simulink model "SPWM_Three_Phase_Three_Level_Inverter"  (R2022a)
settings: Solver=ode4  StartTime=0.0  StopTime=1  FixedStep=1e-5  RelTol=1e-3
libraries: spsIGBTDiodeLib x12, simulink x6, spsSeriesRLCBranchLib x3, spsDCVoltageSourceLib x1, spsGroundLib x1, spsThreePhaseVIMeasurementLib x1, spspowerguiLib x1
settings Model: Creator=nikos  LastModifiedBy=nikos

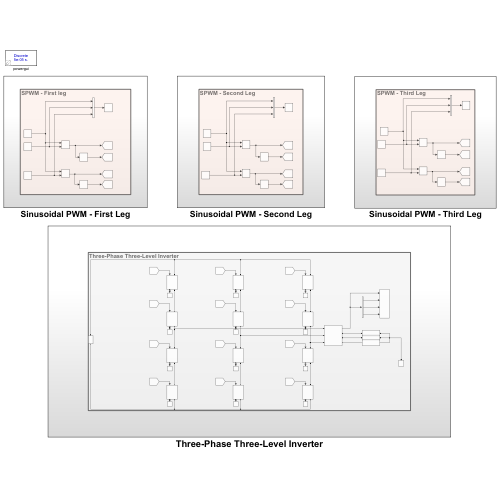
[thumbnail: Simulink's stored preview of the top-level diagram]
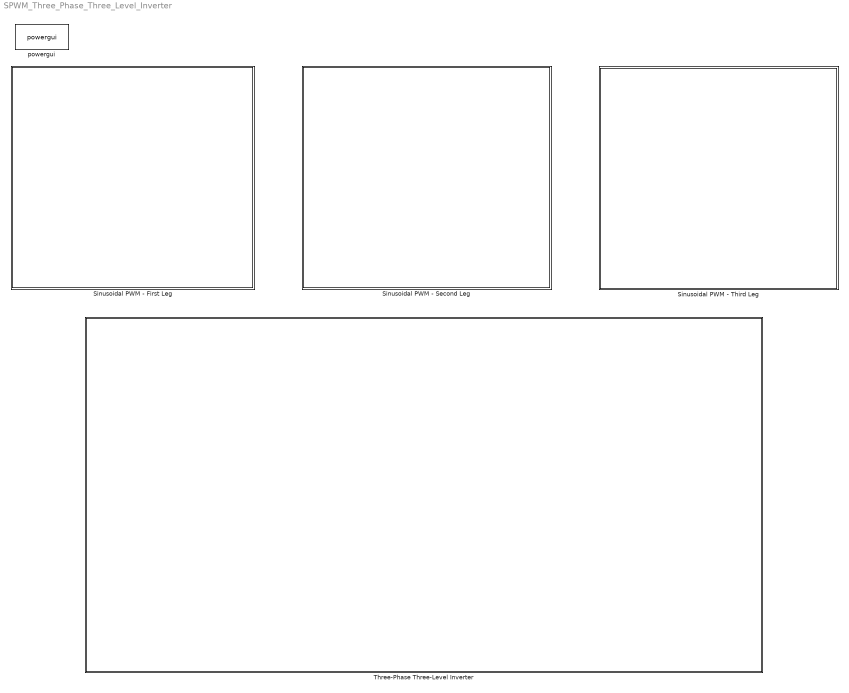
== system SPWM_Three_Phase_Three_Level_Inverter ==
  Sinusoidal PWM - First Leg : Subsystem
  Sinusoidal PWM - Second Leg : Subsystem
  Sinusoidal PWM - Third Leg : Subsystem
  Three-Phase Three-Level Inverter : Subsystem
  powergui : spspowerguiLib/powergui  Priority=1  SimulationMode=Discrete  SampleTime=50e-6  frequency=60  Iterations=50  frequencyindice=0  Pbase=100e6  ErrMax=1e-4  UnitsV=kV  UnitsW=MW  buscounter=0  FunctionMessages=off  echomessages=off  EnableUseOfTLC=off  CurrentSourceSwitches=off  DisableSnubberDevices=off  DisableRonSwitches=off  DisableVfSwitches=off  DisplayEquations=off  AutomaticDiscreteSolvers=off  SolverType=Tustin/Backward Euler (TBE)  Interpol=off  ExternalGateDelay=off  methode=off  Ts=100  x0status=blocks  SPID=on  SwTol=0  HookPort=off  NonlinearTolerance=1e-4  nMaxIteration=100  ContinueOnMaxIteration=off  RestoreLinks=warning  ResistiveCurrentMeasurement=off  Frange=[0:2:500]  Ylog=off  Xlog=on  ShowGrid=off  save=off  variable=ZData  structure=0  ZoomFFT=off  StartTime=0.0  cycles=1  DisplayStyle=1  fundamental=60  FreqAxis=off  MaxFrequency=1000  frequencyindicesteady=1  RmsSteady=1  display=off

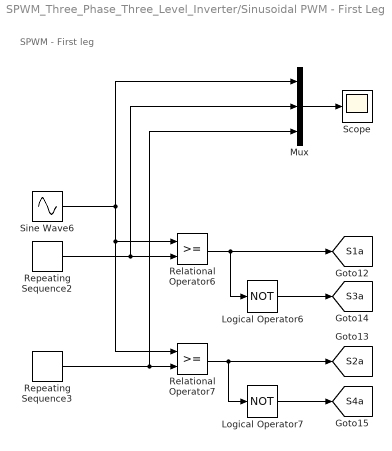
== system SPWM_Three_Phase_Three_Level_Inverter/Sinusoidal PWM - First Leg ==
  note: SPWM - First leg
  Logical Operator6 : Logic  Operator=NOT  AllPortsSameDT=off  OutDataTypeStr=boolean
  Logical Operator7 : Logic  Operator=NOT  AllPortsSameDT=off  OutDataTypeStr=boolean
  Mux : Mux  Inputs=3
  Relational Operator6 : RelationalOperator  OutDataTypeStr=boolean  RndMeth=Simplest  InputSameDT=off
  Relational Operator7 : RelationalOperator  OutDataTypeStr=boolean  RndMeth=Simplest  InputSameDT=off
  Repeating Sequence2 : simulink/Sources/Repeating Sequence  rep_seq_t=[0 1 2]/10000  rep_seq_y=[0 1 0]
  Repeating Sequence3 : simulink/Sources/Repeating Sequence  rep_seq_t=[0 1 2]/10000  rep_seq_y=[-1 0 -1]
  Scope : Scope
  Sine Wave6 : Sin  Frequency=2*pi*50  SampleTime=0
  tag scope: S1a=global, S2a=global, S3a=global, S4a=global
  wires:
  Mux/1 -> Scope/1
  Repeating Sequence2/1 -> Mux/2, Relational Operator6/2
  Sine Wave6/1 -> Mux/1, Relational Operator6/1, Relational Operator7/1
  Logical Operator7/1 -> [S4a]
  Repeating Sequence3/1 -> Mux/3, Relational Operator7/2
  Relational Operator6/1 -> [S1a], Logical Operator6/1
  Relational Operator7/1 -> Logical Operator7/1, [S2a]
  Logical Operator6/1 -> [S3a]

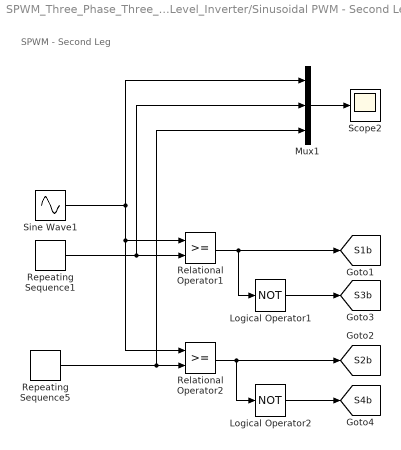
== system SPWM_Three_Phase_Three_Level_Inverter/Sinusoidal PWM - Second Leg ==
  note: SPWM - Second Leg
  Logical Operator1 : Logic  Operator=NOT  AllPortsSameDT=off  OutDataTypeStr=boolean
  Logical Operator2 : Logic  Operator=NOT  AllPortsSameDT=off  OutDataTypeStr=boolean
  Mux1 : Mux  Inputs=3
  Relational Operator1 : RelationalOperator  OutDataTypeStr=boolean  RndMeth=Simplest  InputSameDT=off
  Relational Operator2 : RelationalOperator  OutDataTypeStr=boolean  RndMeth=Simplest  InputSameDT=off
  Repeating Sequence1 : simulink/Sources/Repeating Sequence  rep_seq_t=[0 1 2]/10000  rep_seq_y=[0 1 0]
  Repeating Sequence5 : simulink/Sources/Repeating Sequence  rep_seq_t=[0 1 2]/10000  rep_seq_y=[-1 0 -1]
  Scope2 : Scope
  Sine Wave1 : Sin  Frequency=2*pi*50  Phase=4*pi/3  SampleTime=0
  tag scope: S1b=global, S2b=global, S3b=global, S4b=global
  wires:
  Logical Operator1/1 -> [S3b]
  Relational Operator2/1 -> [S2b], Logical Operator2/1
  Repeating Sequence1/1 -> Mux1/2, Relational Operator1/2
  Sine Wave1/1 -> Mux1/1, Relational Operator1/1, Relational Operator2/1
  Relational Operator1/1 -> [S1b], Logical Operator1/1
  Logical Operator2/1 -> [S4b]
  Mux1/1 -> Scope2/1
  Repeating Sequence5/1 -> Mux1/3, Relational Operator2/2

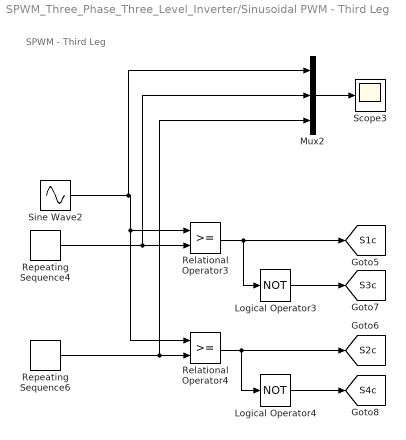
== system SPWM_Three_Phase_Three_Level_Inverter/Sinusoidal PWM - Third Leg ==
  note: SPWM - Third Leg
  Logical Operator3 : Logic  Operator=NOT  AllPortsSameDT=off  OutDataTypeStr=boolean
  Logical Operator4 : Logic  Operator=NOT  AllPortsSameDT=off  OutDataTypeStr=boolean
  Mux2 : Mux  Inputs=3
  Relational Operator3 : RelationalOperator  OutDataTypeStr=boolean  RndMeth=Simplest  InputSameDT=off
  Relational Operator4 : RelationalOperator  OutDataTypeStr=boolean  RndMeth=Simplest  InputSameDT=off
  Repeating Sequence4 : simulink/Sources/Repeating Sequence  rep_seq_t=[0 1 2]/10000  rep_seq_y=[0 1 0]
  Repeating Sequence6 : simulink/Sources/Repeating Sequence  rep_seq_t=[0 1 2]/10000  rep_seq_y=[-1 0 -1]
  Scope3 : Scope
  Sine Wave2 : Sin  Frequency=2*pi*50  Phase=2*pi/3  SampleTime=0
  tag scope: S1c=global, S2c=global, S3c=global, S4c=global
  wires:
  Relational Operator3/1 -> Logical Operator3/1, [S1c]
  Repeating Sequence6/1 -> Mux2/3, Relational Operator4/2
  Mux2/1 -> Scope3/1
  Relational Operator4/1 -> Logical Operator4/1, [S2c]
  Repeating Sequence4/1 -> Mux2/2, Relational Operator3/2
  Sine Wave2/1 -> Mux2/1, Relational Operator4/1, Relational Operator3/1
  Logical Operator3/1 -> [S3c]
  Logical Operator4/1 -> [S4c]

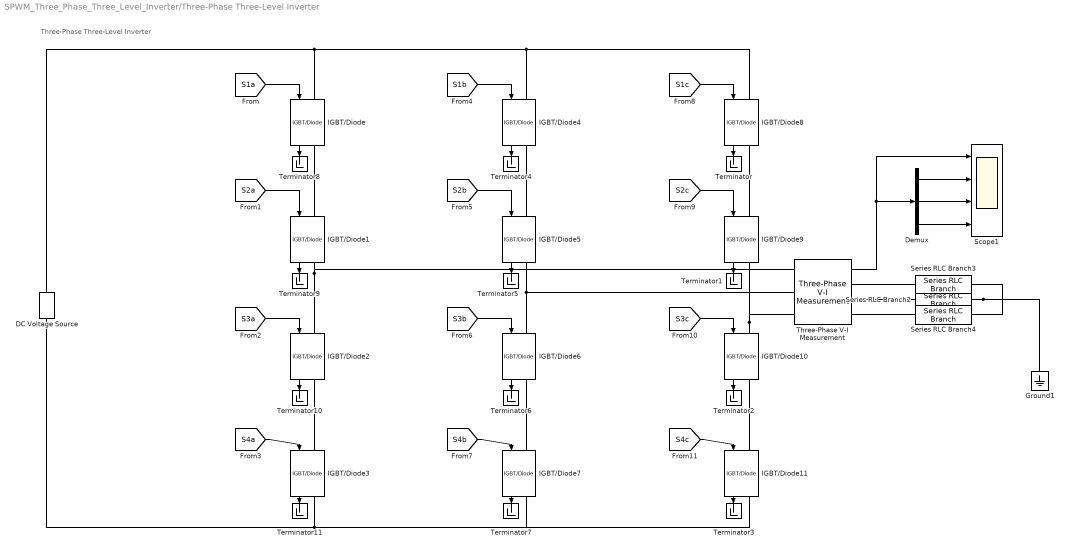
== system SPWM_Three_Phase_Three_Level_Inverter/Three-Phase Three-Level Inverter ==
  note: Three-Phase Three-Level Inverter
  DC Voltage Source : spsDCVoltageSourceLib/DC Voltage Source  Amplitude=100  Measurements=None
  Demux : Demux  Outputs=3
  Ground1 : spsGroundLib/Ground  LConnTagsString=a
  IGBT/Diode{,1..11} (12 alike) : spsIGBTDiodeLib/IGBT//Diode  Ron=1e-3  Rs=1e5  Cs=inf  Measurements=on
  Scope1 : Scope  NumInputPorts=4
  Series RLC Branch2 : spsSeriesRLCBranchLib/Series RLC Branch  LConnTagsString=__new0  RConnTagsString=__new0  BranchType=R  Resistance=100  Inductance=1e-3  SetiL0=off  InitialCurrent=0  Capacitance=1e-6  Setx0=off  InitialVoltage=0  Measurements=None
  Series RLC Branch3 : spsSeriesRLCBranchLib/Series RLC Branch  LConnTagsString=__new0  RConnTagsString=__new0  BranchType=R  Resistance=100  Inductance=1e-3  SetiL0=off  InitialCurrent=0  Capacitance=1e-6  Setx0=off  InitialVoltage=0  Measurements=None
  Series RLC Branch4 : spsSeriesRLCBranchLib/Series RLC Branch  LConnTagsString=__new0  RConnTagsString=__new0  BranchType=R  Resistance=100  Inductance=1e-3  SetiL0=off  InitialCurrent=0  Capacitance=1e-6  Setx0=off  InitialVoltage=0  Measurements=None
  Terminator{,1..11} (12 alike) : Terminator
  Three-Phase V-I Measurement : spsThreePhaseVIMeasurementLib/Three-Phase V-I Measurement  VoltageMeasurement=phase-to-ground  SetLabelV=off  LabelV=Vabc  Vpu=off  VpuLL=off  CurrentMeasurement=no  SetLabelI=off  LabelI=Iabc  Ipu=off  Pbase=100e6  Vbase=500e3  OutputType=Complex  PhasorSimulation=off  PSBequivalent=0
  wires:
  IGBT/Diode8/1 -> Terminator/1
  [S1b] -> IGBT/Diode4/1
  [S2c] -> IGBT/Diode9/1
  [S4b] -> IGBT/Diode7/1
  [S2a] -> IGBT/Diode1/1
  Three-Phase V-I Measurement/1 -> Demux/1, Scope1/1
  [S1c] -> IGBT/Diode8/1
  [S2b] -> IGBT/Diode5/1
  Demux/3 -> Scope1/4
  [S1a] -> IGBT/Diode/1
  IGBT/Diode9/1 -> Terminator1/1
  IGBT/Diode4/1 -> Terminator4/1
  [S4c] -> IGBT/Diode11/1
  IGBT/Diode/1 -> Terminator8/1
  IGBT/Diode10/1 -> Terminator2/1
  Demux/1 -> Scope1/2
  [S3a] -> IGBT/Diode2/1
  IGBT/Diode6/1 -> Terminator6/1
  IGBT/Diode7/1 -> Terminator7/1
  IGBT/Diode2/1 -> Terminator10/1
  IGBT/Diode1/1 -> Terminator9/1
  [S3b] -> IGBT/Diode6/1
  IGBT/Diode11/1 -> Terminator3/1
  Demux/2 -> Scope1/3
  IGBT/Diode5/1 -> Terminator5/1
  [S4a] -> IGBT/Diode3/1
  IGBT/Diode3/1 -> Terminator11/1
  [S3c] -> IGBT/Diode10/1
  connections:
  IGBT/Diode4/RConn1 -- IGBT/Diode5/LConn1
  IGBT/Diode5/RConn1 -- Three-Phase V-I Measurement/LConn2 -- IGBT/Diode6/LConn1
  Series RLC Branch2/LConn1 -- Ground1/LConn1 -- Series RLC Branch4/LConn1 -- Series RLC Branch3/LConn1
  IGBT/Diode2/RConn1 -- IGBT/Diode3/LConn1
  IGBT/Diode10/LConn1 -- Three-Phase V-I Measurement/LConn3 -- IGBT/Diode9/RConn1
  Three-Phase V-I Measurement/RConn2 -- Series RLC Branch2/RConn1
  IGBT/Diode8/LConn1 -- IGBT/Diode4/LConn1 -- DC Voltage Source/RConn1 -- IGBT/Diode/LConn1
  DC Voltage Source/LConn1 -- IGBT/Diode3/RConn1 -- IGBT/Diode7/RConn1 -- IGBT/Diode11/RConn1
  Three-Phase V-I Measurement/LConn1 -- IGBT/Diode1/RConn1 -- IGBT/Diode2/LConn1
  IGBT/Diode10/RConn1 -- IGBT/Diode11/LConn1
  Three-Phase V-I Measurement/RConn3 -- Series RLC Branch4/RConn1
  Three-Phase V-I Measurement/RConn1 -- Series RLC Branch3/RConn1
  IGBT/Diode6/RConn1 -- IGBT/Diode7/LConn1
  IGBT/Diode/RConn1 -- IGBT/Diode1/LConn1
  IGBT/Diode8/RConn1 -- IGBT/Diode9/LConn1
